simulink model "freqdec"  (R2018a)
settings: Solver=FixedStepDiscrete  StartTime=0.0  StopTime=10.0  FixedStep=1e-4  RelTol=1e-3
InitFcn:
  | mbd_pnt_consistency_checks(bdroot(gcs));
undefined symbols (not defined in the file): A11, AN, D10, J, P9, PCR, T12, T13, T6
libraries: mbd_pnt_ec_toolbox x7, simulink x1
settings Model: Creator=oolonthegreat  LastModifiedBy=oolonthegreat
settings DataIOCC: ExternalInput=off  InitialState=off  SaveOutput=off  SignalLogging=off  SaveTime=off
settings OptimizationCC: DefaultParameterBehavior=Inlined  EnhancedBackFolding=on  PassReuseOutputArgsAs=Individual arguments  OptimizeBlockOrder=speed  DifferentSizesBufferReuse=on  OptimizationCustomize=off
settings DebuggingCC: InheritedTsInSrcMsg=none  SingleTaskRateTransMsg=error  ParameterTunabilityLossMsg=error  UnconnectedInputMsg=error  UnconnectedOutputMsg=error  UnconnectedLineMsg=error  UnknownTsInhSupMsg=error
settings HardwareCC: ProdBitPerPointer=32  ProdBitPerSizeT=32  ProdBitPerPtrDiffT=32  ProdLargestAtomicInteger=Long  ProdLargestAtomicFloat=Double  ProdEndianess=BigEndian  ProdWordSize=32  ProdHWDeviceType=Motorola PowerPC
settings SFSimCC: MATLABDynamicMemAlloc=off
settings RTWCC: SystemTargetFile=mbd_pnt.tlc  MakeCommand=mbd_pnt_make_rtw COPY_MDLREF_INCLUDES=0  TemplateMakefile=mbd_pnt.tmf  PostCodeGenCommand=mbd_pnt_analyzegencode(buildInfo)  Description=Model Based Design Toolbox MPC574xP Code Generation Target  GenerateReport=on  IncludeHyperlinkInReport=on  LaunchReport=on  GenerateTraceInfo=on  GenerateTraceReport=on  GenerateTraceReportSl=on  GenerateTraceReportSf=on  GenerateTraceReportEml=on
settings CodeAppCC: ForceParamTrailComments=on  IgnoreCustomStorageClasses=off  OperatorAnnotations=on  SimulinkDataObjDesc=on  SFDataObjDesc=on  InsertBlockDesc=on
settings STFCustomTargetCC: TargetLangStandard=C99 (ISO)  MultiwordLength=256  CombineOutputUpdateFcns=on  SuppressErrorStatus=on  ERTCustomFileBanners=on  SupportContinuousTime=off  SupportNonInlinedSFcns=off  RemoveResetFunc=on  MATLABClassNameForMDSCustomization=Simulink.SoftwareTarget.ERTCustomization  GRTInterface=off  SystemTargetFile=mbd_pnt.tlc
settings ERTTargetCC: TargetLangStandard=C99 (ISO)  ParMdlRefBuildCompliant=off  CompOptLevelCompliant=off  ConcurrentExecutionCompliant=off  SuppressErrorStatus=on  ModelStepFunctionPrototypeControlCompliant=off  CPPClassGenCompliant=off  UseToolchainInfoCompliant=off  InlinedParameterPlacement=NonHierarchical  ERTCustomFileTemplate=example_file_process.tlc

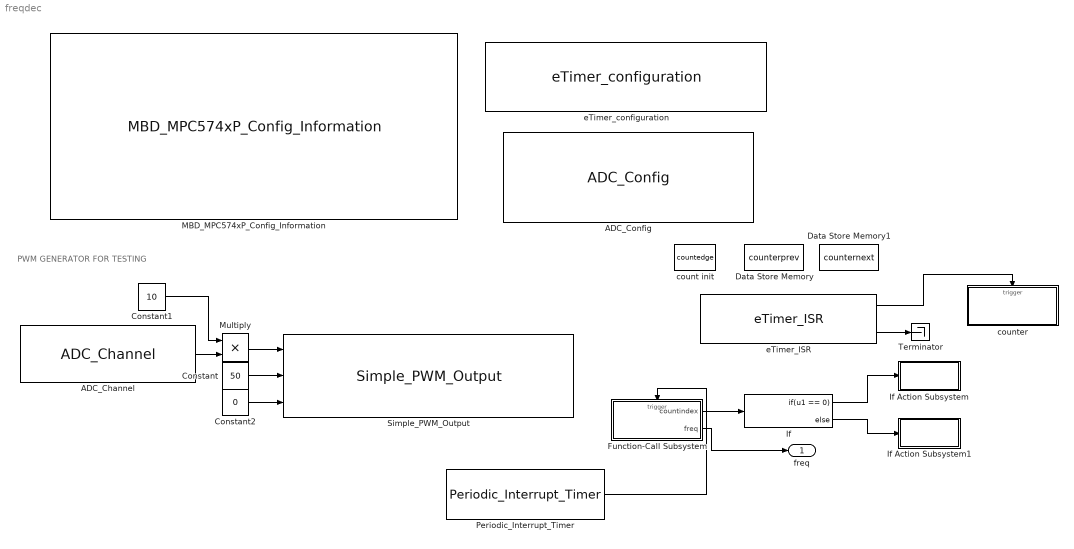
== system freqdec ==
  note: PWM GENERATOR FOR TESTING
  ADC_Channel : mbd_pnt_ec_toolbox/MPC574xP/Motor Control Blocks/ADC_Channel  adc_unit=1  adc_chan0=PCR[71] : E[7] : 48 : 56 : T6 : AN[6]  adc_chan1=PCR[76] : E[12] : 67 : 78 : T12 : AN[6]  adc_chan2=PCR[150] : J[6] : [---] : 65 : P9 : AN[1]  adc_chan3=PCR[64] : E[0] : 68 : 79 : T13 : AN[4]  simulate=off  interrupt=off  adc_mode=Normal  adc_presample=off  pcrNum=76
      settings: SourceProductName=Model Based Design Toolbox for MPC574xP
  ADC_Config : mbd_pnt_ec_toolbox/MPC574xP/Motor Control Blocks/ADC_Config  adc_unit=1  adc_ctu=off  adc_owr=on  adc_wls=0: Left  adc_clk=on  adc_ack=on  adc_edglev=0: Edge  adc_trgen=off  adc_edge=off  adc_ctr0_samp=22  adc_ctr1_samp=11  adc_pscr_preval0=00: AGND_3V  adc_pscr_preconv=off  adc_calbist_admode=110: 12-bit operating mode (high accuracy)  adc_calbist_tsamp=00: 22 cycles of ADC clk  adc_calbist_nrsmpl=01: 32 samples  adc_calbist_avgen=on
      settings: SourceProductName=Model Based Design Toolbox for MPC574xP
  Constant : Constant  Value=50  OutDataTypeStr=uint32
  Constant1 : Constant  Value=10  OutDataTypeStr=uint16
  Constant2 : Constant  Value=0  OutDataTypeStr=uint32
  Data Store Memory : DataStoreMemory  DataStoreName=counterprev  ReadBeforeWriteMsg=warning  WriteAfterWriteMsg=warning  WriteAfterReadMsg=warning  ShowAdditionalParam=off  OutDataTypeStr=double
  Data Store Memory1 : DataStoreMemory  DataStoreName=counternext  ReadBeforeWriteMsg=warning  WriteAfterWriteMsg=warning  WriteAfterReadMsg=warning  ShowAdditionalParam=off  OutDataTypeStr=double
  Function-Call Subsystem : Subsystem  TreatAsAtomicUnit=on
  If : If  IfExpression=u1 == 0
  If Action Subsystem : Subsystem  TreatAsAtomicUnit=on
  If Action Subsystem1 : Subsystem  TreatAsAtomicUnit=on
  MBD_MPC574xP_Config_Information : mbd_pnt_ec_toolbox/MPC574xP/MBD_MPC574xP_Config_Information  disp_str=|  config_params=[]
      | System Clock : 200 MHz
      | Target : MPC5744P
      | Package : 144LQFP
      | XTAL Freq : 40 MHz
      | Compiler : S32 Design Studio
      | Target Type : FLASH
      | Global Interrupt Priority : 8
      | System Tick Interrupt Priority : 12
      | Freemaster : Serial1 (115200 Kbits)
      | Download Code after build : (COM5,115200)
      settings: SourceProductName=Model Based Design Toolbox for MPC574xP
  Multiply : Product  OutDataTypeStr=uint32
  Periodic_Interrupt_Timer : mbd_pnt_ec_toolbox/MPC574xP/Utility Blocks/Periodic_Interrupt_Timer  pit_chan=1  pit_timeout=1000  int_priority=15  pit_timeout_val=49999999
      settings: SourceProductName=Model Based Design Toolbox for MPC574xP
  Simple_PWM_Output : mbd_pnt_ec_toolbox/MPC574xP/Motor Control Blocks/Simple_PWM_Output  pwmModule=0  pwmMod=0  SubModule=0  subMod=0  InitFreq=5000  resolution=1 %  resValue=1  InitDutyA=50  InitDutyB=0  align=center aligned  PhaseShift_A=0  PhaseShift_B=0  Phase_A=0  Phase_B=0  centered=1  doubleSw=off  DoubleS=0  debugSw=off  debug_mode=0  pin0_A0=11: A11 : [120] : [149] : [D10]  pin0_B0=None  pin0_X0=None  pin0_A1=None  pin0_B1=None  pin0_X1=None  pin0_A2=None  pin0_B2=None  pin0_X2=None  pin0_A3=None  pin0_B3=None  pin0_X3=None  pin1_A0=None  pin1_B0=None  pin1_X0=None  pin1_A1=None  pin1_B1=None  pin1_X1=None  pin1_A2=None  pin1_B2=None  pin1_X2=None  pin1_A3=None  pin1_B3=None  pin1_X3=None  pin2_A0=None  pin2_B0=None  pin2_X0=None  pin2_A1=None  pin2_B1=None  pin2_X1=None  pin2_A2=None  pin2_B2=None  pin2_X2=None  pin2_A3=None  pin2_B3=None  pin2_X3=None  pcrNumA=11  pcrNumB=255  pcrNumX=255  polA=off  polB=off  polX=off  octrl=0  syncFrom0=off  masterSync=0  outVal0=off  outVal1=off  outVal2=off  outVal3=off  outVal4=off  outVal5=off  outTrig=0
      settings: SourceProductName=Model Based Design Toolbox for MPC574xP
  Terminator : Terminator
  count init : DataStoreMemory  DataStoreName=countedge  ReadBeforeWriteMsg=warning  WriteAfterWriteMsg=warning  WriteAfterReadMsg=warning  ShowAdditionalParam=off  OutDataTypeStr=double
  counter : Subsystem  TreatAsAtomicUnit=on
  eTimer_ISR : mbd_pnt_ec_toolbox/MPC574xP/Motor Control Blocks/eTimer_ISR  SubModule=0  Timerchan=0  subMod=0  channel=0  isrPriority=14  isrPrio=14
      settings: SourceProductName=Model Based Design Toolbox for MPC574xP
  eTimer_configuration : mbd_pnt_ec_toolbox/MPC574xP/Motor Control Blocks/eTimer_configuration  SubModule=0  TimerChan=0  subMod=0  channel=0  CountMode=001 - Count rising edges of primary source  CNTMODE=1  CountOnce=0 - Count repeatedly  ONCE=0  CountLength=0 - Continue counting to roll over  LENGTH=0  CountDirection=0 - Count up  DIR=0  OutputEnable=0 - The external pin is configured as an input  OEN=0  CoChanInit=00 - Other channels cannot force re-initialization of this channel  COINIT=0  StopAction=0 - Output enable is unaffected by stop mode  STPEN=0  ReloadOnCapt=01 - Reload the counter on a capture 1 event  ROC=1  PrimarySource=11111 - IP Bus clock divide by 128 prescaler  PRISRC=31  PrimSrcPol=0 - True polarity  PIPS=0  SecondarySource=00000 - Counter #0 input pin  SECSRC=0  SecSrcPol=0 - True polarity  SIPS=0  FILT_CNT=0  FILT_PER=0  FILT=0  OutputMode=0000 - Software controlled  OUTMODE=0  OutputPol=0 - True polarity  OPS=0  MasterMode=0 - Disable broadcast of this channel output  MSTR=0  ForcedOutVal=0  VAL=0  CoForce=0 - Other channels cannot force this channel output  COFRC=0  CompLoad1=000 - COMP1 is never preload  CLC1=0  CompLoad2=000 - COMP2 is never preload  CLC2=0  CompareMode="00 - COMP1 and COMP2  are used when the counter is counting up"  CMPMODE=0  CaptMode1=10 - Capture rising edges  CPT1MODE=2  CaptMode2=00 - Capture disabled  CPT2MODE=0  OneShCaptMode=0 - Free running mode is selected  ONESHOT=0  CaptFIFO=0  CFWM=0  CNTRinit=0  COMP1init=0  COMP2init=0  mod0ch0pin="0     : A0   :  [73]   : [86]   : [P12]  input/output"  mod0ch1pin=None  mod0ch2pin=None  mod0ch3pin=None  mod0ch4pin=None  mod0ch5pin=None  mod1ch0pin=None  mod1ch1pin=None  mod1ch2pin=None  mod1ch3pin=None  mod1ch4pin=None  mod1ch5pin=None  mod2ch0pin=None  mod2ch1pin=None  mod2ch2pin=None  mod2ch3pin=None  mod2ch4pin=None  mod2ch5pin=None  pcrNum0=0  pcrNum1=255  pcrNum2=255  pcrNum3=255  pcrNum4=255  pcrNum5=255  TCFIE=off  TCF1IE=off  TCF2IE=off  TOFIE=off  IELFIE=off  IEHFIE=off  ICF1IE=on  ICF2IE=off  INTDMA=64
      settings: SourceProductName=Model Based Design Toolbox for MPC574xP
  freq : Outport
  wires:
  Constant/1 -> Simple_PWM_Output/2
  Constant2/1 -> Simple_PWM_Output/3
  eTimer_ISR/2 -> Terminator/1
  eTimer_ISR/1 -> counter/Trigger
  Periodic_Interrupt_Timer/1 -> Function-Call Subsystem/Trigger
  Function-Call Subsystem/1(countindex) -> If/1
  If/1 -> If Action Subsystem/Action
  If/2 -> If Action Subsystem1/Action
  Function-Call Subsystem/2(freq) -> freq/1
  Multiply/1 -> Simple_PWM_Output/1
  Constant1/1 -> Multiply/1
  ADC_Channel/1 -> Multiply/2

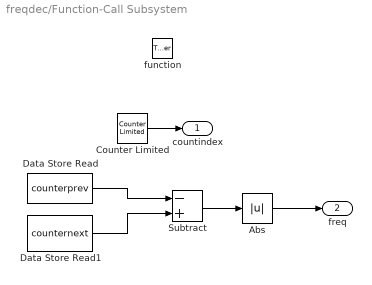
== system freqdec/Function-Call Subsystem ==
  function : TriggerPort  TriggerType=function-call  VariantControl=Variant
  Abs : Abs
  Counter Limited : simulink/Sources/Counter Limited  uplimit=1  tsamp=-1
  Data Store Read : DataStoreRead  DataStoreName=counterprev
  Data Store Read1 : DataStoreRead  DataStoreName=counternext
  Subtract : Sum  Inputs=-+
  countindex : Outport
  freq : Outport  Port=2
  wires:
  Counter Limited/1 -> countindex/1
  Data Store Read/1 -> Subtract/1
  Data Store Read1/1 -> Subtract/2
  Subtract/1 -> Abs/1
  Abs/1 -> freq/1

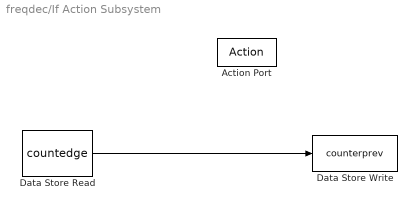
== system freqdec/If Action Subsystem ==
  Action Port : ActionPort  ActionType=then
  Data Store Read : DataStoreRead  DataStoreName=countedge
  Data Store Write : DataStoreWrite  DataStoreName=counterprev
  wires:
  Data Store Read/1 -> Data Store Write/1

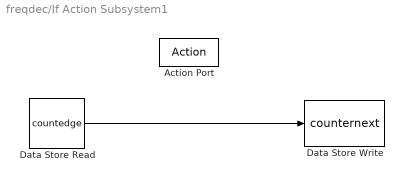
== system freqdec/If Action Subsystem1 ==
  Action Port : ActionPort  ActionType=else
  Data Store Read : DataStoreRead  DataStoreName=countedge
  Data Store Write : DataStoreWrite  DataStoreName=counternext
  wires:
  Data Store Read/1 -> Data Store Write/1

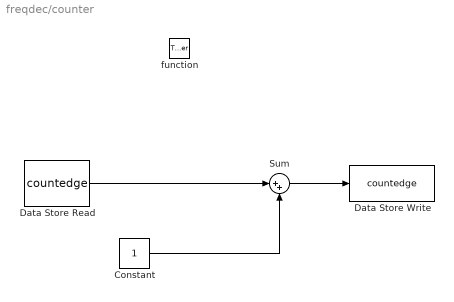
== system freqdec/counter ==
  function : TriggerPort  TriggerType=function-call  VariantControl=Variant
  Constant : Constant  OutDataTypeStr=double
  Data Store Read : DataStoreRead  DataStoreName=countedge
  Data Store Write : DataStoreWrite  DataStoreName=countedge
  Sum : Sum  Inputs=|++
  wires:
  Constant/1 -> Sum/2
  Data Store Read/1 -> Sum/1
  Sum/1 -> Data Store Write/1
